simulink model "Model_1"  (R2020b)
settings: Solver=VariableStepAuto  StartTime=0.0  StopTime=10.0  RelTol=1e-3
settings Model: Creator=Diwakar Reddy  LastModifiedBy=Diwakar Reddy

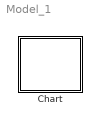
== system Model_1 ==
  Chart : Stateflow chart  TreatAsAtomicUnit=on

== stateflow chart Model_1/Chart ==
  state state1
    entry:
    x=0;
    y=0;
    z=0;
  state state2
    entry:
    y=0;
    z=0;
    x=1;
  state state3
    entry:
    z=0;
    y=1;
    x=0;
  state state4
    entry:
    z=0;
    y=1;
    x=1;
  state state5
    entry:
    z=1;
    y=0;
    x=0;
  (default) -> state1
  state5 -> state1 : [z==1 && y==0 && x==0]
  state1 -> state2 : [z==0 && y==0 && x==0]
  state2 -> state3 : [z==0 && y==0 && x==1]
  state3 -> state4 : [z==0 && y==1 && x==0]
  state4 -> state5 : [z==0 && y==1 && x==1]
